simulink model "TJA1042_Loop_Example"  (R2024a)
settings: Solver=FixedStepAuto  StartTime=0.0  StopTime=10.0  RelTol=1e-3
PreLoadFcn:
  | % NXP_MBDT_S32K3 callback: DO NOT REMOVE
  | mbd_s32k3.common.nxp.model_callbacks.preLoadFcn();
PostLoadFcn:
  | % NXP_MBDT_S32K3 callback: DO NOT REMOVE
  | mbd_s32k3.common.nxp.model_callbacks.postLoadFcn();
InitFcn:
  | % NXP_MBDT_S32K3 callback: DO NOT REMOVE
  | mbd_s32k3.common.nxp.model_callbacks.initFcn();
undefined symbols (not defined in the file or in its folder): mbd_s32k3
libraries: mbd_s32k3_communication_library x7, mbd_s32k3_io_library x5, mbd_s32k3_isr_library x1
(part 2 of 5)

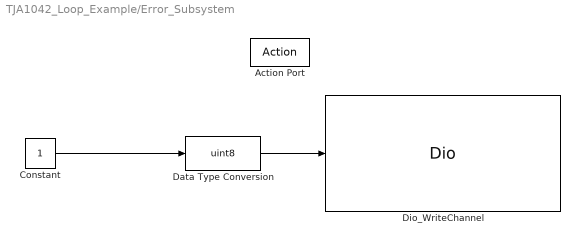
== system TJA1042_Loop_Example/Error_Subsystem ==
  Action Port : ActionPort  ActionPortLabel=if(u1 ~= 0)
  Constant : Constant  OutDataTypeStr=Inherit: Inherit via back propagation
  Data Type Conversion : DataTypeConversion  OutDataTypeStr=uint8  SaturateOnIntegerOverflow=off  RndMeth=Floor
  Dio_WriteChannel : mbd_s32k3_io_library/Dio  api_func=Dio_WriteChannel  channel=RGBLED0_RED  channel_group=No channel groups configured  port=PTA_H  gpioSim=on  text=<binary blob, 4382 chars, not shown>
      settings: SourceProductName=IO Blocks
  wires:
  Constant/1 -> Data Type Conversion/1
  Data Type Conversion/1 -> Dio_WriteChannel/1
